simulink model "ImageTest"  (R2018b)
settings: Solver=FixedStepAuto  StartTime=0.0  StopTime=inf  RelTol=1e-3
PreLoadFcn:
  | % ROS setup
  | rosshutdown;
  | ipAddr = '';
  | rosinit(ipAddr)
  | 
  | % Sample times
  | sampleTime = 0.2;
model workspace (MAT data in the model file):
  SL_ROS_VariableLengthArrays_MaxSizes.CommonInfo.ArrayTruncateAction = 'EmitWarning'
  SL_ROS_VariableLengthArrays_MaxSizes.MsgTypeMap = containers.Map
  SL_ROS_VariableLengthArrays_MaxSizes.MsgTypeMap.serialization.keys = {'sensor_msgs/Image'}
  SL_ROS_VariableLengthArrays_MaxSizes.MsgTypeMap.serialization.values{1}(1).PropertyName = 'Data'
  SL_ROS_VariableLengthArrays_MaxSizes.MsgTypeMap.serialization.values{1}(1).DataType = 'uint8'
  SL_ROS_VariableLengthArrays_MaxSizes.MsgTypeMap.serialization.values{1}(1).MaxLength = 921600
  SL_ROS_VariableLengthArrays_MaxSizes.MsgTypeMap.serialization.values{1}(2).PropertyName = 'Encoding'
  SL_ROS_VariableLengthArrays_MaxSizes.MsgTypeMap.serialization.values{1}(2).DataType = 'uint8'
  SL_ROS_VariableLengthArrays_MaxSizes.MsgTypeMap.serialization.values{1}(2).MaxLength = 128
  SL_ROS_VariableLengthArrays_MaxSizes.MsgTypeMap.serialization.uniformity = 0
  SL_ROS_VariableLengthArrays_MaxSizes.MsgTypeMap.serialization.keyType = 'char'
  SL_ROS_VariableLengthArrays_MaxSizes.MsgTypeMap.serialization.valueType = 'any'
libraries: robotlib x3, visionanalysis x1
settings Model: Creator=The MathWorks, Inc.  LastModifiedBy=carlos6120
settings OptimizationCC: EnhancedBackFolding=on  PassReuseOutputArgsAs=Individual arguments  MaxStackSize=64  OptimizeBlockOrder=speed  DifferentSizesBufferReuse=on  OptimizationCustomize=off
settings DebuggingCC: ParameterTunabilityLossMsg=error  LibraryContextMissingDiagnostic=none
settings HardwareCC: ProdBitPerPointer=32  ProdBitPerSizeT=32  ProdBitPerPtrDiffT=32  ProdLargestAtomicFloat=None  ProdIntDivRoundTo=Undefined  ProdEndianess=Unspecified  ProdWordSize=32  ProdHWDeviceType=Generic->Unspecified (assume 32-bit Generic)
settings SFSimCC: SimUseLocalCustomCode=off  MATLABDynamicMemAlloc=off
settings RTWCC: SystemTargetFile=ert.tlc  HardwareBoard=Robot Operating System (ROS)  TLCOptions="-aInlineSetEventsForThisBaseRateFcn=TLC_FALSE -aSuppressMultiTaskScheduler=TLC_FALSE  -aRateBasedStepFcn=0"  TemplateMakefile=ert_default_tmf  GenerateReport=on  RTWUseLocalCustomCode=off  Toolchain=Catkin  IncludeHyperlinkInReport=on  LaunchReport=on  TargetLang=C++  GenerateTraceInfo=on  GenerateTraceReport=on  GenerateTraceReportSl=on  GenerateTraceReportSf=on  GenerateTraceReportEml=on
settings CodeAppCC: ForceParamTrailComments=on  IgnoreCustomStorageClasses=off  OperatorAnnotations=on  SimulinkDataObjDesc=on  SFDataObjDesc=on  InsertBlockDesc=on

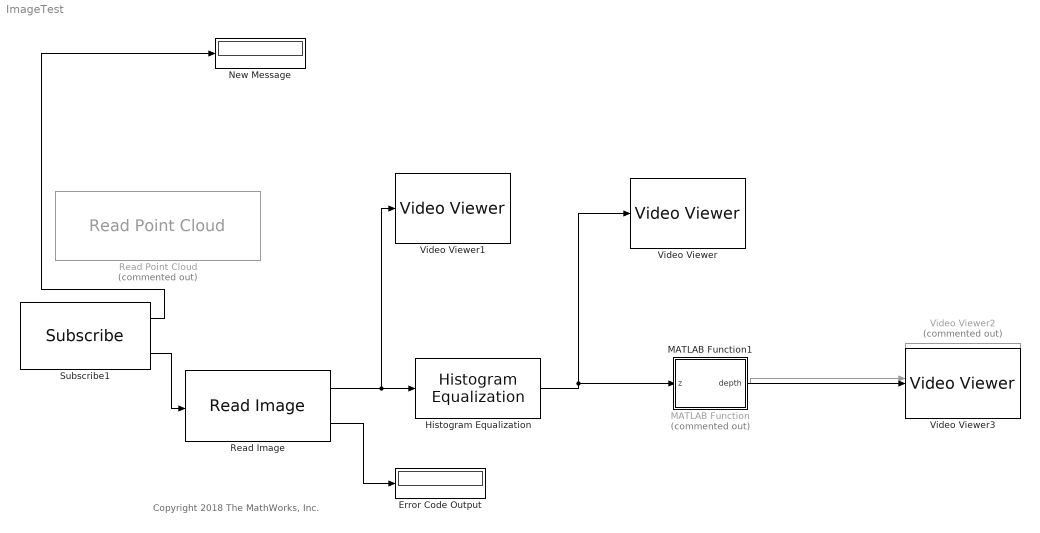
== system ImageTest ==
  note: Copyright 2018 The MathWorks, Inc.
  Error Code Output : Display
  Histogram Equalization : visionanalysis/Histogram Equalization  specify=Uniform  numbins=64  src=Specify via dialog  hist=ones(1,64)
      settings: SourceProductName=Computer Vision System Toolbox  SourceProductBaseCode=VP
  MATLAB Function : MATLAB Function  Commented=on  TreatAsAtomicUnit=on
  MATLAB Function1 : MATLAB Function  TreatAsAtomicUnit=on
  New Message : Display
  Read Image : robotlib/Read Image  MaximumImageSize=[480, 640]  ImageEncoding=16uc1  ShowAlphaOutput=off  ShowErrorCodeOutput=on  VariableSizeOutputs=off
      settings: SourceProductName=Robotics System Toolbox  SourceProductBaseCode=RO
  Read Point Cloud : robotlib/Read Point Cloud  Commented=on  MaximumPointCloudSize=[ 480, 640 ]  PreserveStructure=off  ShowRGBOutput=off  ShowIntensityOutput=off  ShowErrorCodeOutput=on  VariableSizeOutputs=off
      settings: SourceProductName=Robotics System Toolbox  SourceProductBaseCode=RO
  Subscribe1 : robotlib/Subscribe  topicSource=Select from ROS network  topic=/camera/depth/image_rect_raw  messageType=sensor_msgs/Image  sampleTime=-1  messageQueueLength=1
      settings: SourceProductBaseCode=RO
  Video Viewer : VideoViewer  FigPos=[554 815 573 353]
  Video Viewer1 : VideoViewer  FigPos=[981 938 901 592]
  Video Viewer2 : VideoViewer  Commented=on  FigPos=[887 783 583 383]
  Video Viewer3 : VideoViewer  FigPos=[887 783 583 383]
  wires:
  Read Image/2 -> Error Code Output/1
  Read Image/1 -> Video Viewer1/1, Histogram Equalization/1
  Subscribe1/2 -> Read Image/1
  Subscribe1/1 -> New Message/1
  Histogram Equalization/1 -> MATLAB Function/1(z), Video Viewer/1
  MATLAB Function/1(depth) -> Video Viewer2/1
  MATLAB Function1/1(depth) -> Video Viewer3/1

== matlab function ImageTest/MATLAB Function1 ==
  data: z input uint16; depth output uint16 size=[480,640] [..307200]
function depth = SimpleKalman(z)
%
%
% persistent A H Q R
% persistent x P
% persistent firstRun 
% 
% persistent I J 
% persistent M N


[M,N] = size(z);

depth = zeros(M,N);

if isempty (firstRun)
    A = 1;
    H = 1;

    Q = 0;
    R = 4;

    x = 0;
    P = 6;

    firstRun = 1;
end
% x=uint16(x);

for I=1:M
    for J = 1:N
%         z = z(I,J);
        xp = A*x;
        Pp = A*P*A'+Q;

        K = Pp*H'/(H*Pp*H'+R);

        x= xp+K*(z-H*xp);
        P = Pp-K*H*Pp;
        depth(I,J) = x;
    end
end

== matlab function ImageTest/MATLAB Function ==
  data: z input; depth output uint16 size=[480,640] [..307200]
function depth = SimpleKalman(z)
%
%
% uint16 A H Q R
% persistent x P
% persistent firstRun 
% 
% persistent I J 
% persistent M N


[M,N] = size(z);

depth = zeros(M,N);

if isempty (firstRun)
    A = 1;
    H = 1;

    Q = 0;
    R = 4;

    x = 0;
    P = 6;

    firstRun = 1;
end
% x=uint16(x);

for I=1:M
    for J = 1:N
%         z = z(I,J);
        xp = A*x;
        Pp = A*P*A'+Q;

        K = Pp*H'/(H*Pp*H'+R);

        x= xp+K*(z-H*xp);
        P = Pp-K*H*Pp;
        depth(I,J) = x;
    end
end
